simulink model "S4"  (R2023b)
settings: Solver=FixedStepAuto  StartTime=0.0  StopTime=10  FixedStep=Step_T  RelTol=1e-3
values from neighbouring files (symbols this model uses):
  x_1_0 = 0.2    [P_sim.m]
  x_2_0 = 0.5    [P_sim.m]
  x_3_0 = -1    [P_sim.m]
settings Model: Creator=admin  LastModifiedBy=admin

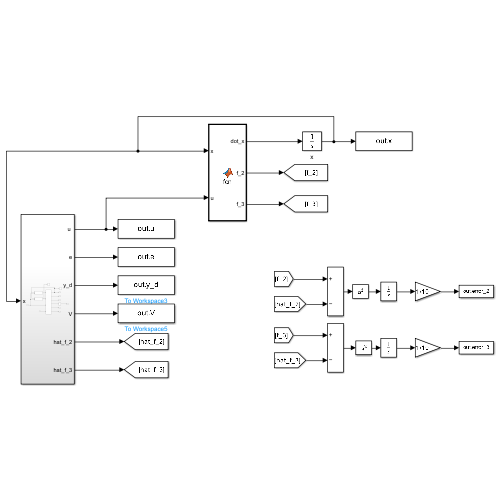
[thumbnail: Simulink's stored preview of the top-level diagram]
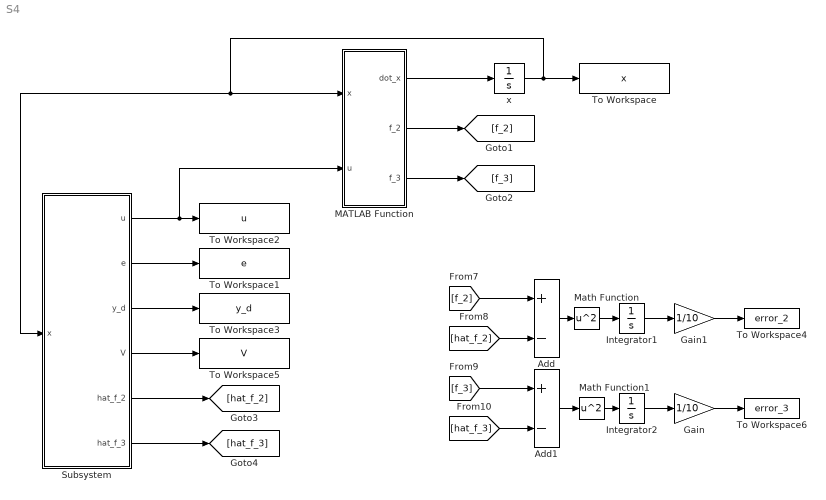
== system S4 ==
  Add : Sum  Inputs=+-
  Add1 : Sum  Inputs=+-
  Gain : Gain  Gain=1/10
  Gain1 : Gain  Gain=1/10
  Integrator1 : Integrator
  Integrator2 : Integrator
  MATLAB Function : MATLAB Function  TreatAsAtomicUnit=on
  Math Function : Math  Operator=square
  Math Function1 : Math  Operator=square
  Subsystem : Subsystem
  To Workspace : ToWorkspace  VariableName=x  SaveFormat=Timeseries  SampleTime=-1
  To Workspace1 : ToWorkspace  VariableName=e  SaveFormat=Timeseries  SampleTime=-1
  To Workspace2 : ToWorkspace  VariableName=u  SaveFormat=Timeseries  SampleTime=-1
  To Workspace3 : ToWorkspace  VariableName=y_d  SaveFormat=Timeseries  SampleTime=-1
  To Workspace4 : ToWorkspace  VariableName=error_2  SaveFormat=Timeseries  SampleTime=-1
  To Workspace5 : ToWorkspace  VariableName=V  SaveFormat=Timeseries  SampleTime=-1
  To Workspace6 : ToWorkspace  VariableName=error_3  SaveFormat=Timeseries  SampleTime=-1
  x : Integrator  InitialCondition=[x_1_0;x_2_0;x_3_0]
  wires:
  MATLAB Function/1(dot_x) -> x/1
  x/1 -> To Workspace/1, MATLAB Function/1(x), Subsystem/1(x)
  Subsystem/1("u ") -> MATLAB Function/2(u), To Workspace2/1
  Subsystem/2(e) -> To Workspace1/1
  Subsystem/3(y_d) -> To Workspace3/1
  Subsystem/4(V) -> To Workspace5/1
  MATLAB Function/2(f_2) -> [f_2]
  MATLAB Function/3(f_3) -> [f_3]
  Math Function1/1 -> Integrator2/1
  [f_3] -> Add1/1
  Gain/1 -> To Workspace6/1
  Gain1/1 -> To Workspace4/1
  Math Function/1 -> Integrator1/1
  [hat_f_3] -> Add1/2
  [hat_f_2] -> Add/2
  [f_2] -> Add/1
  Integrator1/1 -> Gain1/1
  Integrator2/1 -> Gain/1
  Add/1 -> Math Function/1
  Add1/1 -> Math Function1/1
  Subsystem/5(hat_f_2) -> [hat_f_2]
  Subsystem/6(hat_f_3) -> [hat_f_3]

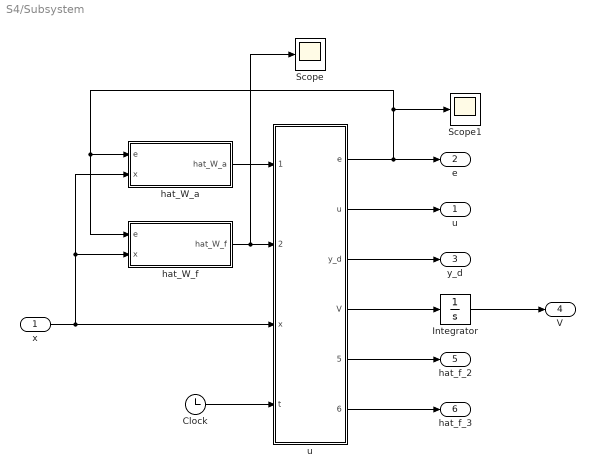
== system S4/Subsystem ==
  x : Inport
  Clock : Clock
  Integrator : Integrator
  Scope : Scope
  Scope1 : Scope
  hat_W_a : Subsystem
  hat_W_f : Subsystem
  u : MATLAB Function  TreatAsAtomicUnit=on
  "u " : Outport
  e : Outport  Port=2
  y_d : Outport  Port=3
  V : Outport  Port=4
  hat_f_2 : Outport  Port=5
  hat_f_3 : Outport  Port=6
  wires:
  u/2(u) -> "u "/1
  Clock/1 -> u/4(t)
  u/1(e) -> e/1, Scope1/1, hat_W_a/1(e), hat_W_f/1(e)
  u/3(y_d) -> y_d/1
  hat_W_f/1(hat_W_f) -> Scope/1, u/2(hat_W_f)
  hat_W_a/1(hat_W_a) -> u/1(hat_W_a)
  x/1 -> hat_W_a/2(x), hat_W_f/2(x), u/3(x)
  Integrator/1 -> V/1
  u/4(V) -> Integrator/1
  u/5(hat_f_2) -> hat_f_2/1
  u/6(hat_f_3) -> hat_f_3/1

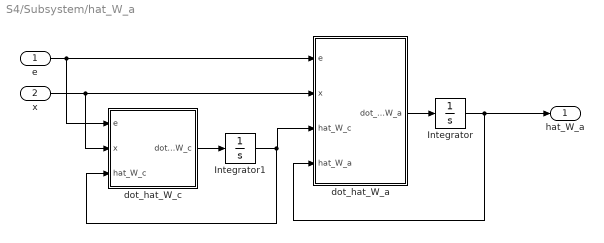
== system S4/Subsystem/hat_W_a ==
  e : Inport
  x : Inport  Port=2
  Integrator : Integrator
  Integrator1 : Integrator
  dot_hat_W_a : MATLAB Function  TreatAsAtomicUnit=on
  dot_hat_W_c : MATLAB Function  TreatAsAtomicUnit=on
  hat_W_a : Outport
  wires:
  dot_hat_W_a/1(dot_hat_W_a) -> Integrator/1
  Integrator/1 -> dot_hat_W_a/4(hat_W_a), hat_W_a/1
  e/1 -> dot_hat_W_a/1(e), dot_hat_W_c/1(e)
  x/1 -> dot_hat_W_a/2(x), dot_hat_W_c/2(x)
  dot_hat_W_c/1(dot_hat_W_c) -> Integrator1/1
  Integrator1/1 -> dot_hat_W_c/3(hat_W_c), dot_hat_W_a/3(hat_W_c)

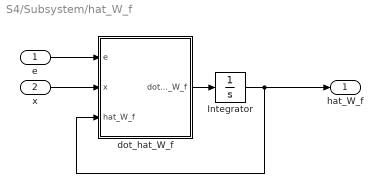
== system S4/Subsystem/hat_W_f ==
  e : Inport
  x : Inport  Port=2
  Integrator : Integrator
  dot_hat_W_f : MATLAB Function  TreatAsAtomicUnit=on
  hat_W_f : Outport
  wires:
  dot_hat_W_f/1(dot_hat_W_f) -> Integrator/1
  Integrator/1 -> dot_hat_W_f/3(hat_W_f), hat_W_f/1
  e/1 -> dot_hat_W_f/1(e)
  x/1 -> dot_hat_W_f/2(x)

== matlab function S4/Subsystem/u ==
  data: e output size=[3,1]; hat_W_a input; hat_W_f input; x input size=[3,1]; t input; u output; pam parameter; y_d output size=1; V output size=1; hat_f_2 output; hat_f_3 output
function [e,u,y_d,V,hat_f_2,hat_f_3]  = fcn(hat_W_a,hat_W_f,x,t,pam)

y_d = sin(t);
dot_y_d = cos(t);

lambda_1=6;
lambda_2=15;
lambda_3=10;

x_1 = x(1);
x_2 = x(2);
x_3 = x(3);

hat_W_a_1 = hat_W_a(:,1);
hat_W_a_2 = hat_W_a(:,2);
hat_W_a_3 = hat_W_a(:,3);

hat_W_f_1 = hat_W_f(:,1);
hat_W_f_2 = hat_W_f(:,2);
hat_W_f_3 = hat_W_f(:,3);

%% 第一阶
e_1 = x_1 - y_d;

S_f1 = RBF_based(x_1);
S_j1 = RBF_based([x_1;e_1]);

alpha_1 = -lambda_1*e_1-hat_W_f_1'*S_f1-hat_W_a_1'*S_j1+dot_y_d;
 
%% 第二阶
e_2 = x_2 - alpha_1;

S_f2 = RBF_based([x_1;x_2]);
S_j2 = RBF_based([x_1;x_2;e_2]);

alpha_2 = -lambda_2*e_2-hat_W_f_2'*S_f2-hat_W_a_2'*S_j2;

%% 第三阶
e_3 = x_3 - alpha_2;

S_f3 = RBF_based([x_1;x_2;x_3]);
S_j3 = RBF_based([x_1;x_2;x_3;e_3]);

u = -lambda_3*e_3-hat_W_f_3'*S_f3-hat_W_a_3'*S_j3;

e = [e_1;e_2;e_3];

V = e_1^2+u^2;

hat_f_2 = hat_W_f_2'*S_f2;
hat_f_3 = hat_W_f_3'*S_f3;

== matlab function S4/MATLAB Function ==
  data: x input; dot_x output; u input; pam parameter; f_2 output; f_3 output
function [dot_x,f_2,f_3]  = fcn(x,u,pam)

x_1 = x(1);
x_2 = x(2);
x_3 = x(3);

dot_x_1 = x_2;
dot_x_2 = x_3+pam.M/pam.D*sin(x_1)-pam.B/pam.D*x_2;
dot_x_3 = u+pam.K_m/pam.L*x_2-pam.J/pam.L*x_3;

dot_x = [dot_x_1;dot_x_2;dot_x_3];
f_2 = pam.M/pam.D*sin(x_1)-pam.B/pam.D*x_2;
f_3 = pam.K_m/pam.L*x_2-pam.J/pam.L*x_3;

== matlab function S4/Subsystem/hat_W_f/dot_hat_W_f ==
  data: e input; x input; dot_hat_W_f output size=[24,3]; hat_W_f input
function dot_hat_W_f = fcn(e,x,hat_W_f)

x_1 = x(1);
x_2 = x(2);
x_3 = x(3);

e_1 = e(1);
e_2 = e(2);
e_3 = e(3);

hat_W_f_1 = hat_W_f(:,1);
hat_W_f_2 = hat_W_f(:,2);
hat_W_f_3 = hat_W_f(:,3);

%% 第一阶
S_f_1 = RBF_based(x_1);
dot_hat_W_f_1 = 1*(S_f_1*e_1-1*hat_W_f_1);
 
%% 第二阶
S_f_2 = RBF_based([x_1;x_2]);
dot_hat_W_f_2 = 1*(S_f_2*e_2-1*hat_W_f_2);

%% 第三阶
S_f_3 = RBF_based([x_1;x_2;x_3]);
dot_hat_W_f_3 = 1*(S_f_3*e_3-1*hat_W_f_3);

dot_hat_W_f = [dot_hat_W_f_1,dot_hat_W_f_2,dot_hat_W_f_3];

== matlab function S4/Subsystem/hat_W_a/dot_hat_W_a ==
  data: e input; x input; hat_W_c input; dot_hat_W_a output size=[24,3]; hat_W_a input
function dot_hat_W_a = fcn(e,x,hat_W_c,hat_W_a)

x_1 = x(1);
x_2 = x(2);
x_3 = x(3);

e_1 = e(1);
e_2 = e(2);
e_3 = e(3);

hat_W_a_1 = hat_W_a(:,1);
hat_W_a_2 = hat_W_a(:,2);
hat_W_a_3 = hat_W_a(:,3);

hat_W_c_1 = hat_W_c(:,1);
hat_W_c_2 = hat_W_c(:,2);
hat_W_c_3 = hat_W_c(:,3);

%% 第一阶
S_j1 = RBF_based([x_1;e_1]);
dot_hat_W_a_1 = -S_j1*S_j1'*(5*(hat_W_a_1-hat_W_c_1)+5*hat_W_c_1);
 
%% 第二阶
S_j2 = RBF_based([x_1;x_2;e_2]);
dot_hat_W_a_2 = -S_j2*S_j2'*(5*(hat_W_a_2-hat_W_c_2)+5*hat_W_c_2);

%% 第三阶
S_j3 = RBF_based([x_1;x_2;x_3;e_3]);
dot_hat_W_a_3 = -S_j2*S_j2'*(5*(hat_W_a_2-hat_W_c_2)+5*hat_W_c_2);

dot_hat_W_a = [dot_hat_W_a_1,dot_hat_W_a_2,dot_hat_W_a_3];

== matlab function S4/Subsystem/hat_W_a/dot_hat_W_c ==
  data: e input; x input; hat_W_c input size=[24,3]; dot_hat_W_c output
function dot_hat_W_c = fcn(e,x,hat_W_c)

x_1 = x(1);
x_2 = x(2);
x_3 = x(3);

e_1 = e(1);
e_2 = e(2);
e_3 = e(3);

hat_W_c_1 = hat_W_c(:,1);
hat_W_c_2 = hat_W_c(:,2);
hat_W_c_3 = hat_W_c(:,3);

%% 第一阶
S_j1 = RBF_based([x_1;e_1]);
dot_hat_W_c_1 = -5*S_j1*S_j1'*hat_W_c_1;
 
%% 第二阶
S_j2 = RBF_based([x_1;x_2;e_2]);
dot_hat_W_c_2 = -5*S_j2*S_j2'*hat_W_c_2;

%% 第三阶
S_j3 = RBF_based([x_1;x_2;x_3;e_3]);
dot_hat_W_c_3 = -5*S_j3*S_j3'*hat_W_c_3;

dot_hat_W_c = [dot_hat_W_c_1,dot_hat_W_c_2,dot_hat_W_c_3];
